simulink model "sl_subsys_enabtrig1"  (Simulink 6.0)
settings: Solver=FixedStepDiscrete  SolverMode=SingleTasking  StartTime=0.0  StopTime=25  FixedStep=.25  RelTol=1e-3
settings Model: CovMetricSettings=d  Creator=The MathWorks Inc.  LastModifiedBy=batserve  ExtModeAutoUpdateStatusClock=off
settings OptimizationCC: BlockReduction=off  BooleanDataType=off
settings DebuggingCC: CheckExecutionContextPreStartOutputMsg=on  CheckExecutionContextRuntimeOutputMsg=on  SolverPrmCheckMsg=none
settings HardwareCC: TargetUnknown=on

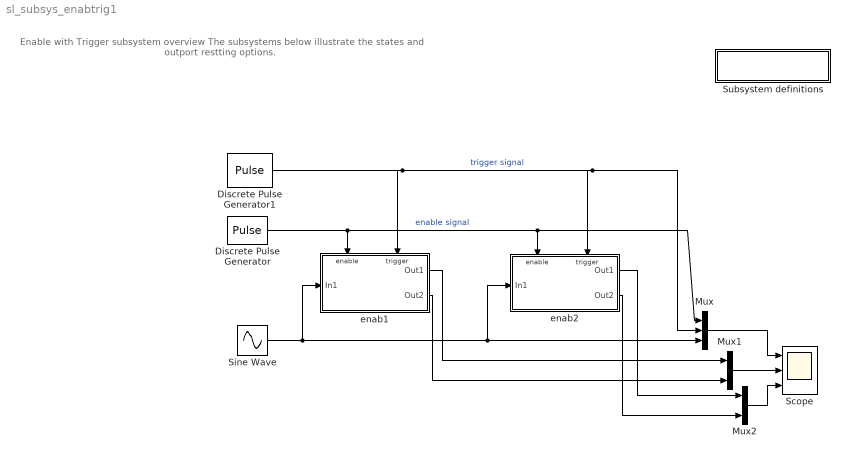
== system sl_subsys_enabtrig1 ==
  note: Enable with Trigger subsystem overview
      |
      | The subsystems below illustrate the states and outport
      | restting options.
  " Subsystem definitions" : Subsystem  PropExecContextAcrossSSBoundary=on
      settings: OpenFcn=helpview([matlabroot,'/toolbox/simulink/simdemos/sl_subsys_definitions.html']);
      mask Display: disp('Subsystem\ndefinitions')
  Discrete Pulse Generator : DiscretePulseGenerator  Period=20  PulseWidth=10  SampleTime=.25
  Discrete Pulse Generator1 : DiscretePulseGenerator  SampleTime=.25
  Mux : Mux  Inputs=3
  Mux1 : Mux  Inputs=2
  Mux2 : Mux  Inputs=2
  Scope : Scope  NumInputPorts=3
      settings: TimeRange=25  YMin=-5~-5~-5  YMax=5~5~5
  Sine Wave : Sin  SineType=Sample based  Amplitude=2  Samples=20  SampleTime=.25
  enab1 : Subsystem  TreatAsAtomicUnit=on  PropExecContextAcrossSSBoundary=on
  enab2 : Subsystem  TreatAsAtomicUnit=on  PropExecContextAcrossSSBoundary=on
  wires:
  enab1/1(Out1) -> Mux1/1
  enab2/1(Out1) -> Mux2/1
  Discrete Pulse Generator/1 -> enab2/Enable, Mux/1, enab1/Enable  "enable signal"
  Sine Wave/1 -> enab1/1(In1), enab2/1(In1), Mux/3
  Mux/1 -> Scope/1
  Mux1/1 -> Scope/2
  enab1/2(Out2) -> Mux1/2
  Mux2/1 -> Scope/3
  enab2/2(Out2) -> Mux2/2
  Discrete Pulse Generator1/1 -> enab1/Trigger, enab2/Trigger, Mux/2  "trigger signal"

== system sl_subsys_enabtrig1/ Subsystem definitions ==

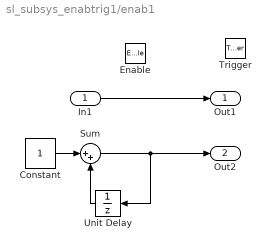
== system sl_subsys_enabtrig1/enab1 ==
  In1 : Inport  Port=1  LatchInput=off
  Enable : EnablePort  StatesWhenEnabling=reset
      settings: AttributesFormatString=States when enabling = %<StatesWhenEnabling>
  Trigger : TriggerPort
  Constant : Constant
  Sum : Sum  Inputs=|++  SaturateOnIntegerOverflow=on  InputSameDT=on
  Unit Delay : UnitDelay  Orientation=left  SampleTime=-1
  Out1 : Outport  OutputWhenDisabled=reset  InitialOutput=5
      settings: AttributesFormatString=IC=%<InitialOutput>\nOutput when disabled=%<OutputWhenDisabled>
  Out2 : Outport  Port=2
      settings: AttributesFormatString=IC = %<InitialOutput>\nOutput when disabled = %<OutputWhenDisabled>
  wires:
  In1/1 -> Out1/1
  Sum/1 -> Out2/1, Unit Delay/1
  Constant/1 -> Sum/1
  Unit Delay/1 -> Sum/2

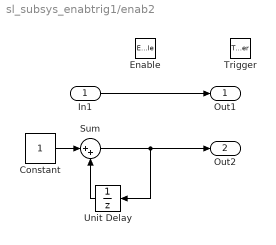
== system sl_subsys_enabtrig1/enab2 ==
  In1 : Inport  Port=1  LatchInput=off
  Enable : EnablePort
      settings: AttributesFormatString=States when enabling = %<StatesWhenEnabling>
  Trigger : TriggerPort
  Constant : Constant
  Sum : Sum  Inputs=|++  SaturateOnIntegerOverflow=on  InputSameDT=on
  Unit Delay : UnitDelay  Orientation=left  SampleTime=-1
  Out1 : Outport  InitialOutput=1
      settings: AttributesFormatString=IC=%<InitialOutput>\nOutput when disabled=%<OutputWhenDisabled>
  Out2 : Outport  Port=2
      settings: AttributesFormatString=IC = %<InitialOutput>\nOutput when disabled = %<OutputWhenDisabled>
  wires:
  Unit Delay/1 -> Sum/2
  Constant/1 -> Sum/1
  Sum/1 -> Unit Delay/1, Out2/1
  In1/1 -> Out1/1
